simulink model "v2_sim_LQI_ideal"  (R2023b)
settings: Solver=VariableStepAuto  StartTime=0.0  StopTime=15  RelTol=1e-10
undefined symbols (not defined in the file or in its folder): K
settings Model: Creator=kiraa  LastModifiedBy=kiraa

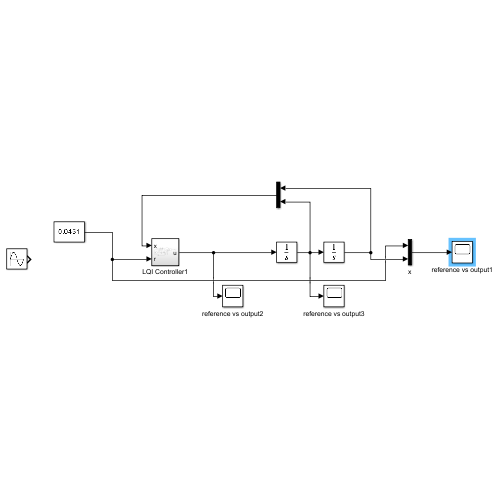
[thumbnail: Simulink's stored preview of the top-level diagram]
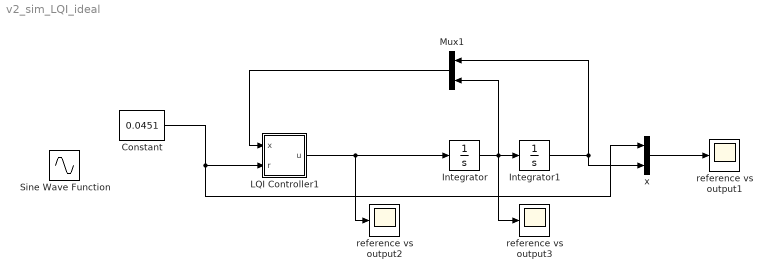
== system v2_sim_LQI_ideal ==
  Constant : Constant  Value=0.0451
  Integrator : Integrator
  Integrator1 : Integrator  InitialCondition=0.1
  LQI Controller1 : Subsystem
  Mux1 : Mux  Inputs=2
  Sine Wave Function : Sin  Amplitude=0.005  Bias=0.0451  Frequency=0.3  SampleTime=0
  reference vs output1 : Scope
  reference vs output2 : Scope
  reference vs output3 : Scope
  x : Mux  Inputs=2
  wires:
  Mux1/1 -> LQI Controller1/1(x)
  Integrator/1 -> reference vs output3/1, Mux1/2, Integrator1/1
  Integrator1/1 -> Mux1/1, x/2
  Constant/1 -> x/1, LQI Controller1/2(r)
  x/1 -> reference vs output1/1
  LQI Controller1/1(u) -> Integrator/1, reference vs output2/1

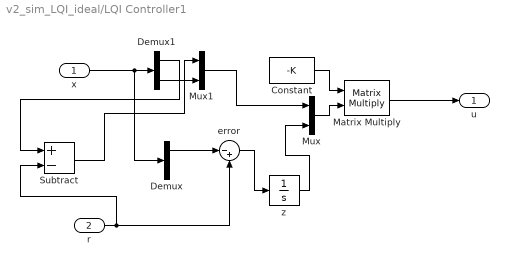
== system v2_sim_LQI_ideal/LQI Controller1 ==
  x : Inport
  r : Inport  Port=2
  Constant : Constant  Value=-K  VectorParams1D=off
  Demux : Demux  Outputs=2
  Demux1 : Demux  Outputs=2
  Matrix Multiply : Product  Multiplication=Matrix(*)
  Mux : Mux  Inputs=2
  Mux1 : Mux  Inputs=2
  Subtract : Sum  Inputs=+-
  error : Sum  Inputs=|-+
  z : Integrator  InitialCondition=0.1
  u : Outport
  wires:
  Constant/1 -> Matrix Multiply/1
  Matrix Multiply/1 -> u/1
  x/1 -> Demux1/1, Demux/1
  Mux/1 -> Matrix Multiply/2
  z/1 -> Mux/2
  Demux/1 -> error/1
  error/1 -> z/1
  Demux1/2 -> Mux1/2
  Demux1/1 -> Subtract/1
  Mux1/1 -> Mux/1
  r/1 -> Subtract/2, error/2
  Subtract/1 -> Mux1/1
